simulink model "motor"  (R2024a)
settings: Solver=ode45  StartTime=0.0  StopTime=1  RelTol=1e-4
values from neighbouring files (symbols this model uses):
  B = 0.1    [set_DC_motor_param.m]
  J = .00252    (= 0.00252)    [set_DC_motor_param.m]
  K = Te_rated/Ia_rated    (= 0.424752712124)    [set_DC_motor_param.m]
  Kac = 1/Kpc    (= 0.235294117647)    [set_DC_motor_param.m]
  Kas = 1/Kps    (= 84.2763317706)    [set_DC_motor_param.m]
  Kic = Ra*Wcc    (= 650)    [set_DC_motor_param.m]
  Kis = J*Wcs*Wcs/(5*Te_rated)    (= 0.118657276485)    [set_DC_motor_param.m]
  Kpc = La*Wcc    (= 4.25)    [set_DC_motor_param.m]
  Kps = J*Wcs/Te_rated    (= 0.0118657276485)    [set_DC_motor_param.m]
  La = 1.7e-3    (= 0.0017)    [set_DC_motor_param.m]
  Ra = 0.26    [set_DC_motor_param.m]
  Te_lim_k = 1    [set_DC_motor_param.m]
  Te_rated = Power/Wm_rated    (= 10.6188178031)    [set_DC_motor_param.m]
  Va_rated = 140    [set_DC_motor_param.m]
settings Model: Creator=CDSL-2  LastModifiedBy=CDSL-2

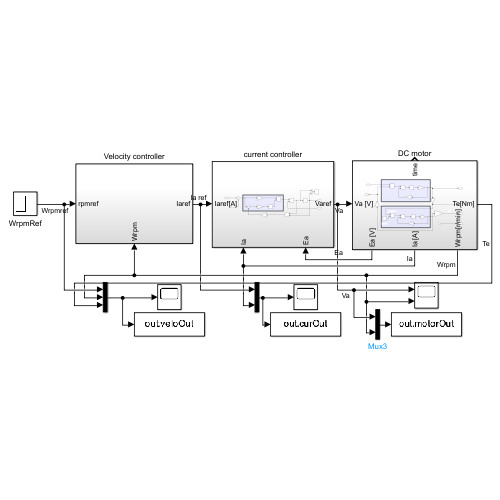
[thumbnail: Simulink's stored preview of the top-level diagram]
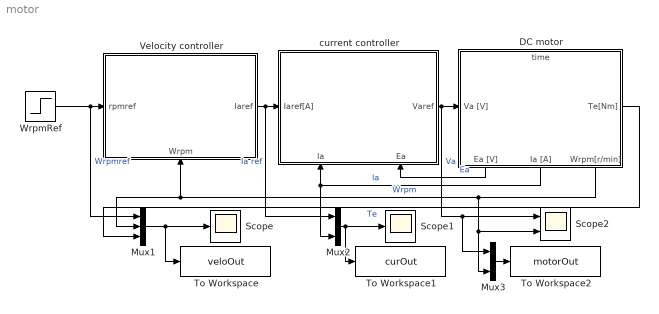
== system motor ==
  DC motor : Subsystem
      settings: PortSchema="{\"entries\":[{\"content\":{\"sides\":[{\"content\":{\"connectorIds\":[\"In1\"]},\"type\":\"ConnectorPlacement.EquallySpacedRectSide\",\"uuid\":\"85d4c81a-2654-4ec9-b469-a8d409c866cc\"},{\"content\":{\"connectorIds\":[\"Out1\"],\"side\":\"RIGHT\"},\"type\":\"ConnectorPlacement.EquallySpacedRectSide\",\"uuid\":\"d9a934b4-e029-4d73-8471-bbe711fb3a53\"},{\"content\":{\"connectorIds\":[\"Out5\"],\"side\":\"TOP\"},\"type\":\"ConnectorPlacement.EquallySpacedRectSide\",\"uuid\":\"d9616158-b721-4b6e-9bc7-8ae67fbd09b9\"},{\"content\":{\"connectorIds\":[\"Out2\",\"Out3\",\"Out4\"],\"side\":\"BOTTOM\"},\"type\":\"ConnectorPlacement.EquallySpacedRectSide\",\"uuid\":\"58ad4a41-e3b9-4acb-83d1-554c4d521999\"}]},\"type\":\"ConnectorPlacement.EquallySpacedConnector\",\"uuid\":\"4cedf73e-3f54-46ef-8108-6c91f544ad78\"}],\"packageUris\":[\"http://schema.mathworks.com/mf0/Connector/R2020b\"],\"version\":\"1.0\"}"
  Mux1 : Mux  Inputs=3
  Mux2 : Mux  Inputs=2
  Mux3 : Mux  Inputs=2
  Scope : Scope
  Scope1 : Scope
  Scope2 : Scope  NumInputPorts=2
  To Workspace : ToWorkspace  VariableName=veloOut  SaveFormat=Timeseries  SampleTime=-1
  To Workspace1 : ToWorkspace  VariableName=curOut  SaveFormat=Timeseries  SampleTime=-1
  To Workspace2 : ToWorkspace  VariableName=motorOut  SaveFormat=Timeseries  SampleTime=-1
  Velocity controller : Subsystem
      settings: PortSchema="{\"entries\":[{\"content\":{\"sides\":[{\"content\":{\"connectorIds\":[\"In1\"]},\"type\":\"ConnectorPlacement.EquallySpacedRectSide\",\"uuid\":\"5eb2e018-7adc-4776-84e2-3754f72fb2b9\"},{\"content\":{\"connectorIds\":[\"Out1\"],\"side\":\"RIGHT\"},\"type\":\"ConnectorPlacement.EquallySpacedRectSide\",\"uuid\":\"2c350664-51fa-477f-b85c-6d22ec9e1a05\"},{\"content\":{\"side\":\"TOP\"},\"type\":\"ConnectorPlacement.EquallySpacedRectSide\",\"uuid\":\"c8ad1243-7e07-4fd2-a383-232e0aaeeba4\"},{\"content\":{\"connectorIds\":[\"In2\"],\"side\":\"BOTTOM\"},\"type\":\"ConnectorPlacement.EquallySpacedRectSide\",\"uuid\":\"57141480-15e7-4b94-afb7-3c913f547fa8\"}]},\"type\":\"ConnectorPlacement.EquallySpacedConnector\",\"uuid\":\"1fc0ef46-6a58-4f46-9e58-7123f91773a0\"}],\"packageUris\":[\"http://schema.mathworks.com/mf0/Connector/R2020b\"],\"version\":\"1.0\"}"
  WrpmRef : Step  Time=0.05  After=500  SampleTime=0
  current controller : Subsystem
      settings: PortSchema="{\"entries\":[{\"content\":{\"sides\":[{\"content\":{\"connectorIds\":[\"In1\"]},\"type\":\"ConnectorPlacement.EquallySpacedRectSide\",\"uuid\":\"cafd2066-022e-4be2-a315-6658f49e1702\"},{\"content\":{\"connectorIds\":[\"Out1\"],\"side\":\"RIGHT\"},\"type\":\"ConnectorPlacement.EquallySpacedRectSide\",\"uuid\":\"e39f233d-5bd3-4f8b-9519-c23b51301a08\"},{\"content\":{\"side\":\"TOP\"},\"type\":\"ConnectorPlacement.EquallySpacedRectSide\",\"uuid\":\"c76cc58b-c96d-4471-94fb-46c95a5dd2e8\"},{\"content\":{\"connectorIds\":[\"In2\",\"In3\"],\"side\":\"BOTTOM\"},\"type\":\"ConnectorPlacement.EquallySpacedRectSide\",\"uuid\":\"45048253-9aa8-4e2e-9d07-f0d42f53913a\"}]},\"type\":\"ConnectorPlacement.EquallySpacedConnector\",\"uuid\":\"73e078e2-0cae-4c03-beac-d2866033d42a\"}],\"packageUris\":[\"http://schema.mathworks.com/mf0/Connector/R2020b\"],\"version\":\"1.0\"}"
  wires:
  DC motor/2(Ea [V]) -> current controller/3(Ea)  "Ea"
  DC motor/3(Ia [A]) -> Mux2/2, current controller/2(Ia)  "Ia"
  current controller/1(Varef) -> Mux3/1, Scope2/1, DC motor/1(Va [V])  "Va"
  WrpmRef/1 -> Mux1/1, Velocity controller/1(rpmref)  "Wrpmref"
  Velocity controller/1(Iaref) -> Mux2/1, current controller/1(Iaref[A])  "Ia ref"
  DC motor/4(Wrpm[r/min]) -> Scope2/2, Mux3/2, Mux1/2, Velocity controller/2(Wrpm)  "Wrpm"
  Mux1/1 -> To Workspace/1, Scope/1
  Mux2/1 -> To Workspace1/1, Scope1/1
  Mux3/1 -> To Workspace2/1
  DC motor/1(Te[Nm]) -> Mux1/3  "Te"

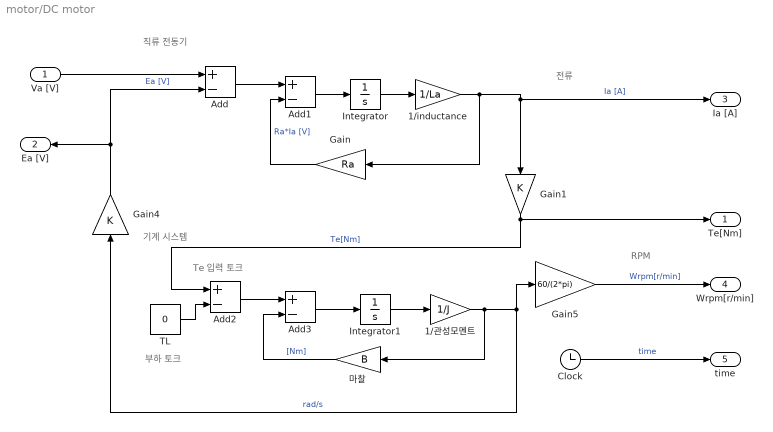
== system motor/DC motor ==
  note: 직류 전동기
  note: 기계 시스템
  note: Te 입력 토크
  note: 전류
  note: RPM
  note: 부하 토크
  Va [V] : Inport
  1/inductance : Gain  Gain=1/La
  1/관성모멘트 : Gain  Gain=1/J
  Add{,1..3} (4 alike) : Sum  Inputs=+-
  Clock : Clock
  Gain : Gain  Gain=Ra
  Gain1 : Gain  Gain=K
  Gain4 : Gain  Gain=K
  Gain5 : Gain  Gain=60/(2*pi)
  Integrator : Integrator
  Integrator1 : Integrator
  TL : Constant  Value=0
  마찰 : Gain  Gain=B
  Te[Nm] : Outport
  Ea [V] : Outport  Port=2
  Ia [A] : Outport  Port=3
  Wrpm[r/min] : Outport  Port=4
  time : Outport  Port=5
  wires:
  Gain1/1 -> Te[Nm]/1, Add2/1  "Te[Nm]"
  Gain5/1 -> Wrpm[r/min]/1  "Wrpm[r/min]"
  1/관성모멘트/1 -> Gain4/1, Gain5/1, 마찰/1  "rad/s"
  1/inductance/1 -> Ia [A]/1, Gain1/1, Gain/1  "Ia [A]"
  Add3/1 -> Integrator1/1
  Gain4/1 -> Ea [V]/1, Add/2  "Ea [V]"
  Add2/1 -> Add3/1
  Integrator/1 -> 1/inductance/1
  Va [V]/1 -> Add/1
  Integrator1/1 -> 1/관성모멘트/1
  Add/1 -> Add1/1
  Clock/1 -> time/1  "time"
  TL/1 -> Add2/2
  Gain/1 -> Add1/2  "Ra*Ia [V]"
  마찰/1 -> Add3/2  "[Nm]"
  Add1/1 -> Integrator/1

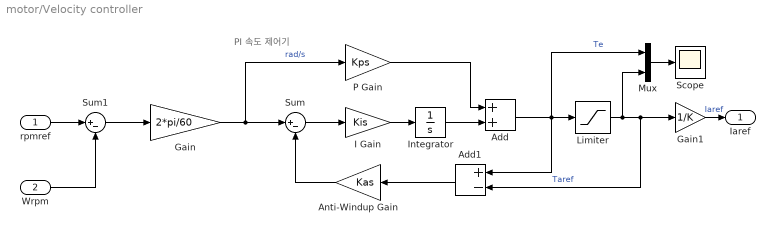
== system motor/Velocity controller ==
  note: PI 속도 제어기
  rpmref : Inport
  Wrpm : Inport  Port=2
  Add : Sum
  Add1 : Sum  Inputs=+-
  Anti-Windup Gain : Gain  Gain=Kas
  Gain : Gain  Gain=2*pi/60
  Gain1 : Gain  Gain=1/K
  I Gain : Gain  Gain=Kis
  Integrator : Integrator
  Limiter : Saturate  UpperLimit=Te_rated*Te_lim_k  LowerLimit=-Te_rated*Te_lim_k
  Mux : Mux  Inputs=2
  P Gain : Gain  Gain=Kps
  Scope : Scope
  Sum : Sum  Inputs=|+-
  Sum1 : Sum  Inputs=|+-
  Iaref : Outport
  wires:
  Add1/1 -> Anti-Windup Gain/1
  P Gain/1 -> Add/1
  Sum/1 -> I Gain/1
  Limiter/1 -> Add1/2, Gain1/1, Mux/2  "Taref"
  Add/1 -> Add1/1, Limiter/1, Mux/1  "Te"
  I Gain/1 -> Integrator/1
  Gain/1 -> P Gain/1, Sum/1  "rad/s"
  Integrator/1 -> Add/2
  Anti-Windup Gain/1 -> Sum/2
  Wrpm/1 -> Sum1/2
  rpmref/1 -> Sum1/1
  Gain1/1 -> Iaref/1  "Iaref"
  Sum1/1 -> Gain/1
  Mux/1 -> Scope/1

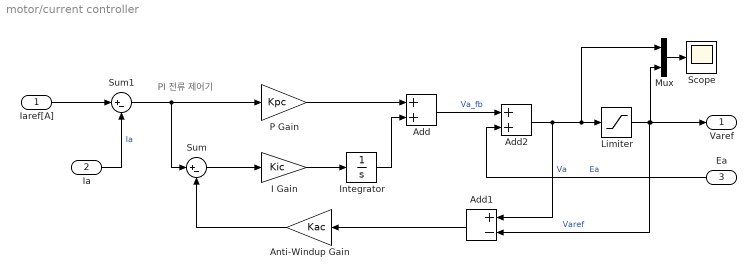
== system motor/current controller ==
  note: PI 전류 제어기
  Iaref[A] : Inport
  Ia : Inport  Port=2
  Ea : Inport  Port=3
  Add : Sum
  Add1 : Sum  Inputs=+-
  Add2 : Sum
  Anti-Windup Gain : Gain  Gain=Kac
  I Gain : Gain  Gain=Kic
  Integrator : Integrator
  Limiter : Saturate  UpperLimit=Va_rated  LowerLimit=-Va_rated
  Mux : Mux  Inputs=2
  P Gain : Gain  Gain=Kpc
  Scope : Scope
  Sum : Sum  Inputs=|+-
  Sum1 : Sum  Inputs=|+-
  Varef : Outport
  wires:
  Sum1/1 -> Sum/1, P Gain/1
  Ea/1 -> Add2/2  "Ea"
  Iaref[A]/1 -> Sum1/1
  Integrator/1 -> Add/2
  Add2/1 -> Mux/1, Limiter/1, Add1/1  "Va"
  Limiter/1 -> Mux/2, Varef/1, Add1/2  "Varef"
  P Gain/1 -> Add/1
  Anti-Windup Gain/1 -> Sum/2
  Sum/1 -> I Gain/1
  Add/1 -> Add2/1  "Va_fb"
  I Gain/1 -> Integrator/1
  Add1/1 -> Anti-Windup Gain/1
  Ia/1 -> Sum1/2  "Ia"
  Mux/1 -> Scope/1
